simulink model "UREC_microgrid"  (R2021b)
settings: Solver=ode23tb  StartTime=0.0  StopTime=length(meters(:, 1))*SecsPerFiveMins  RelTol=1e-3
PostLoadFcn:
  | % EXCEL SCRAPING
  | 
  | [meters, timesdates] = xlsread('ExcelDataMk3.xlsx');
  | %{
  | Format:
  | No column headers
  | Times in 1st column
  | Dates in 2nd column
  | Meter data in columns 2-5
  | Times and dates will become 2 different columns of "timesdates"
  | %}
  | 
  | [pv0_power, pv0_timestamps] = xlsread('PVMk2_0axis.xlsx');
  | %{
  | Format:
  | No column headers
  | Timestamps in 1st column
  | PV output data in 2nd column
  | %}
  | 
  | [pv1_power, pv1_timestamps] = xlsread('PVMk2_1axis.xlsx');
  | %{
  | Format:
  | No column headers
  | Timestamps in 1st column
  | PV output data in 2nd column
  | %}
  | 
  | [pv2_power, pv2_timestamps] = xlsread('PVMk2_2axis.xlsx');
  | %{
  | Format:
  | No column headers
  | Timestamps in 1st column
  | PV output data in 2nd column
  | %}
  | 
  | [wind_power, wind_timestamps] = xlsread('WindMk1.xlsx');
  | %{
  | Format:
  | No column headers
  | Timestamps in 1st column
  | Wind output data in 2nd column
  | %}
  | 
  | 
  | % CONSTANTS
  | 
  | NumBatteryBanks = 1;
  | SecsPerFiveMins = 300;
  | MaxBatteryPower = 1200; %max kW for charge AND discharge of ONE Saft battery
  | TurbinekW = 1600; %The capacity of the wind turbine model, in kW
  | ThreePVs = [pv0_power, pv1_power, pv2_power]; %For easy selection with Dashboard
model workspace (MAT data in the model file):
  PVAxes = 0
  testVal = 1
  testVal1 = 1
  testVal2 = 1
undefined symbols (not defined in the file): meters, pv0_power, wind_power
libraries: simulink x6, exampleMicrogridLibrary x4, spsThreePhaseDynamicLoadLib x3, spsThreePhaseSourceLib x1, spspowerguiLib x1
settings Model: SimulationMode=accelerator  Creator=andre  LastModifiedBy=andre

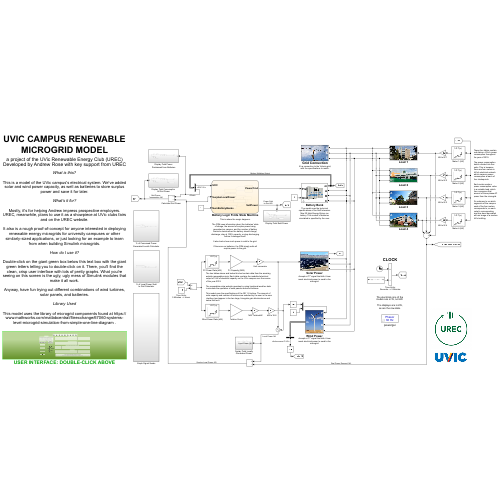
[thumbnail: Simulink's stored preview of the top-level diagram]
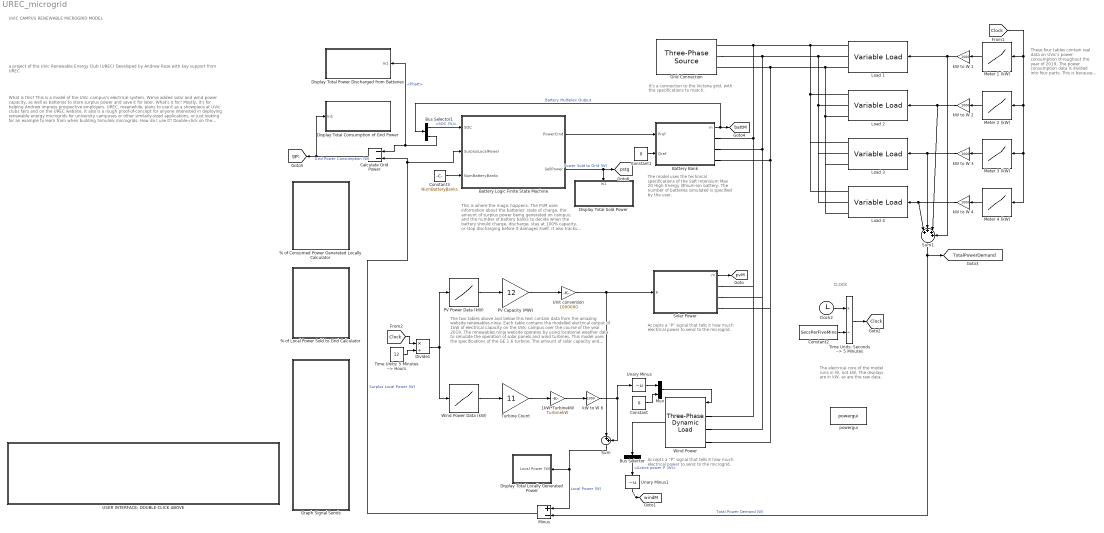
== system UREC_microgrid ==
  note: This is where the magic happens.
      |
      | The FSM uses information about the batteries' state of charge, the amount of surplus power being generated on campus, and the number of battery banks to decide when the battery should charge, discharge, stay at 100% capacity, or stop discharging before it damages itself.
      |
      | It also tracks how much power is sold to the grid.
      |
      | If there are no batteries, the FSM simply sells all surplus power to the grid.
  note: The two tables above and below this text contain data from the amazing website renewables.ninja. Each table contains the modelled electrical output of 1kW of electrical capacity on the UVic campus over the course of the year 2019.
      |
      | The renewables.ninja website operates by using locational weather data to simulate the operation of solar panels and wind turbines.
      |
      | This model uses the specifications of the GE 1.6 turbine. The amount of solar capacity and number of turbines are selected by the user in the user interface (and appear in the two large, triangular gain blocks above and below this text).
  note: Accepts a "P" signal that tells it how much electrical power to send to the microgrid.
  note: The model uses the technical specifications of the Saft Intensium Max 20 High Energy lithium-ion battery. The number of batteries simulated is specified by the user.
  note: These four tables contain real data on UVic's power consumption throughout the year of 2019.
      |
      | The power consumption data is divided into four parts. This is because there are four meters in UVic's electrical network which measure power consumption at each of four chokepoints.
      |
      | Each meter sends a power consumption value to a variable load, which then consumes that amount of three-phase AC power from the microgrid.
      |
      | It's unknown to us which segments of the campus each of the four meters corresponds to, so each meter's corresponding load has been decorated with an image of a random UVic building.
  note: UVIC CAMPUS RENEWABLE
      | MICROGRID MODEL
  note: CLOCK
  note: The electrical core of the
      | model runs in W, not kW.
      |
      | The displays are in kW,
      | as are the raw data.
  note: a project of the UVic Renewable Energy Club (UREC)
      | Developed by Andrew Rose with key support from UREC
  note: What is this?
      |
      | This is a model of the UVic campus's electrical system. We've added solar and wind power capacity, as well as batteries to store surplus power and save it for later.
      |
      | What's it for?
      |
      | Mostly, it's for helping Andrew impress prospective employers. UREC, meanwhile, plans to use it as a showpiece at UVic clubs fairs and on the UREC website.
      |
      | It also is a rough proof-of-concept for anyone interested in deploying renewable energy microgrids for university campuses or other similarly-sized applications, or just looking for an example to learn from when building Simulink microgrids.
      |
      | How do I use it?
      |
      | Double-click on the giant green box below this text box with the giant green letters telling you to double-click on it. There, you'll find the clean, crisp user interface with lots of pretty graphs. What you're seeing on this screen is the ugly, ugly mess of Simulink modules that make it all work.
      |
      | Anyway, have fun trying out different combinations of wind turbines, solar panels, and batteries.
      |
      | Library Used
      |
      | This model uses the library of microgrid components found at https://www.mathworks.com/matlabcentral/fileexchange/67060-systems-level-microgrid-simulation-from-simple-one-line-diagram .
  note: It's a connection to the Victoria grid, with the specifications to match.
  note: Accepts a "P" signal that tells it how much electrical power to send to the microgrid.
  % of Consumed Power Generated Locally Calculator : Subsystem
  % of Local Power Sold to Grid Calculator : Subsystem
  "1kW*TurbinekW " : Gain  Gain=TurbinekW
  Battery Bank : Subsystem  mask(Grid-connected Energy Storage (PQ Model)){Vn=208, Fn=60, PnomkW=MaxBatteryPower*NumBatteryBanks, kWh_Rated=2500*NumBatteryBanks, Efficiency=87.5, LimitVec=[100 10], RechargeSOC=11, Precharge=100, autoRecharge=off, Initial_kWh_pc=80, PQvec=[0 0]}
      mask prompts: Vn "Nominal L-L Voltage [Vrms]"; Fn "Nominal Frequency [Hz]"; PnomkW "Rated Power [kW]"; kWh_Rated "Rated Capacity [kWh]"; Efficiency "Overall System Efficiency [%]"; LimitVec "Upper/Lower Charge Limits [%]"; RechargeSOC "SOC to Recharge [%]"; Precharge "Recharge Rate [% of Rated Power]"; autoRecharge "Enable Auto-Recharge"; Initial_kWh_pc "Initial State-of-Charge [0-100%]"; PQvec "Initial Active/Reactive Cmds"
      mask help:
      | The energy storage block models a generic grid-connected energy storage system (ESS), most commonly a battery system. This is a system-level model that does not contain any power electronics, but is useful for load flow, phasor, and hybrid phasor-EMT simulations. The inputs to this block are the commanded active and reactive power of the ESS. The ESS is assumed to have four quadrent operation.
      |
      | For more detailed ESS models, consider the battery block in the Drives library. Consider using this PQ Model to perform load flow studies and switch to a more detailed model when full EMT studies or more advanced controls are required.
      |
      | Note: The initial active/reactive power commands must be specified for use for Load Flow analysis.
      mask init:
      | % Calculate Initial Conditions
      | Pnom = PnomkW*1e3;
      | P0 = -PQvec(1);  Q0 = -PQvec(2);
      | if abs(P0) > Pnom
      |     P0 = sign(P0)*Pnom;
      | end
      | 
      | % Calculate Q0 given Reactive Power Capability Curve
      | Qlim = sqrt(Pnom^2 - P0^2);
      | if Qlim > abs(Q0)
      |     Q0 = sign(Q0)*Qlim;
      | end
      | 
      | UpChrgLim = LimitVec(1);
      | LowChrgLim = LimitVec(2);
      | if Initial_kWh_pc > UpChrgLim && P0 < 0
      |     P0 = 0; Q0 = 0;
      | elseif Initial_kWh_pc < LowChrgLim && P0 > 0
      |     P0 = 0; Q0 = 0;
      | end
      mask DialogControl Container7 Prompt: Grid Connection Properties
      mask DialogControl Container11 Prompt: Charge/Discharge Controls
      mask DialogControl Container12 Prompt: Initial Conditions
      mask Display:
      | image('$imagefile'); % Use "Edit Image" on toolstrip to change.
      | color('black')
      | port_label('input', 1, 'Pref')
      | port_label('input', 2, 'Qref')
      | port_label('output',1,'m')
      | port_label('Rconn',1,'A')
      | port_label('Rconn',2,'B')
      | port_label('Rconn',3,'C')
  Battery Logic Finite State Machine : Stateflow chart  TreatAsAtomicUnit=on
  Bus Selector : BusSelector  OutputSignals=Active power P (W)
  Bus Selector1 : BusSelector  OutputSignals=SOC (%),Pbatt
  Calculate Grid Power : Sum  Inputs=--
  Clock2 : Clock
      settings: Decimation=1000
  Constant : Constant  Value=0
  Constant1 : Constant  Value=0
  Constant2 : Constant  Value=SecsPerFiveMins
  Constant3 : Constant  Value=NumBatteryBanks
  Display Total Consumption of Grid Power : Subsystem
  Display Total Locally Generated Power : Subsystem
  Display Total Power Discharged from Batteries : Subsystem
  Display Total Sold Power : Subsystem
      settings: PortSchema="{\"entries\":[{\"content\":{\"sides\":[{\"content\":{\"connectorIds\":[]},\"type\":\"ConnectorPlacement.EquallySpacedRectSide\",\"uuid\":\"62bf1daa-ae47-4c4c-bb60-5b8a528187ce\"},{\"content\":{\"connectorIds\":[],\"side\":\"RIGHT\"},\"type\":\"ConnectorPlacement.EquallySpacedRectSide\",\"uuid\":\"b0232ea0-dc8f-4c22-91af-b7339a0b5622\"},{\"content\":{\"connectorIds\":[\"In1\"],\"side\":\"TOP\"},\"type\":\"ConnectorPlacement.EquallySpacedRectSide\",\"uuid\":\"43a34dad-e90c-4708-b85a-e2ed5af34da1\"}]},\"type\":\"ConnectorPlacement.EquallySpacedConnector\",\"uuid\":\"1a3bae20-1562-4c93-80ee-9a5a33e73ad3\"}],\"packageUris\":[\"http://schema.mathworks.com/mf0/Connector/R2020b\"],\"version\":\"1.0\"}"
  Divide1 : Product  Inputs=*/
  Graph Signal Sends : Subsystem
  Grid Connection : spsThreePhaseSourceLib/Three-Phase Source  InternalConnection=Yg  VoltagePhases=off  Voltage=208  PhaseAngle=0  Voltage_phases=[25e3 25e3 25e3]/sqrt(3)  PhaseAngles_phases=[0 -120 +120]  Frequency=60  NonIdealSource=on  SpecifyImpedance=off  Resistance=0  Inductance=0  ShortCircuitLevel=250e6  BaseVoltage=208  XRratio=7  BusType=swing  Pref=10e3  Qref=0  Prefabc=[10e3, 10e3, 10e3]  Qrefabc=[0, 0, 0]  Qmin=-inf  Qmax=inf  mask(Three-Phase Source){}
      mask Display:
      | image('$imagefile'); % Use "Edit Image" on toolstrip to change.
      | color('white')
      | port_label('Rconn',1,'A')
      | port_label('Rconn',2,'B')
      | port_label('Rconn',3,'C')
  Load {1..4} (4 alike) : exampleMicrogridLibrary/Variable Load  Vn=208  Fn=60  PF=1  Load0=200e3  mask(Variable Load (PQ Model)){}
      settings: SourceProductName=Example Microgrid Library
      mask Display:
      | image('$imagefile'); % Use "Edit Image" on toolstrip to change.
      | color('white')
      | port_label('input',1,'Load')
      | port_label('Rconn',1,'A')
      | port_label('Rconn',2,'B')
      | port_label('Rconn',3,'C')
  Meter 1 (kW) : Lookup_n-D  NumberOfTableDimensions=1  BreakpointsForDimension1=[0:length(meters(:, 1))-1]  IndexSearchMethod=Linear search  BeginIndexSearchUsingPreviousIndexResult=on  Table=meters(:, 1)  InterpMethod=Flat  InternalRulePriority=Speed  RndMeth=Simplest  InputSameDT=on
  Meter 2 (kW) : Lookup_n-D  NumberOfTableDimensions=1  BreakpointsForDimension1=[0:length(meters(:, 1))-1]  IndexSearchMethod=Linear search  BeginIndexSearchUsingPreviousIndexResult=on  Table=meters(:, 2)  InterpMethod=Flat  InternalRulePriority=Speed  RndMeth=Simplest  InputSameDT=on
  Meter 3 (kW) : Lookup_n-D  NumberOfTableDimensions=1  BreakpointsForDimension1=[0:length(meters(:, 1))-1]  IndexSearchMethod=Linear search  BeginIndexSearchUsingPreviousIndexResult=on  Table=meters(:, 3)  InterpMethod=Flat  InternalRulePriority=Speed  RndMeth=Simplest  InputSameDT=on
  Meter 4 (kW) : Lookup_n-D  NumberOfTableDimensions=1  BreakpointsForDimension1=[0:length(meters(:, 1))-1]  IndexSearchMethod=Linear search  BeginIndexSearchUsingPreviousIndexResult=on  Table=meters(:, 4)  InterpMethod=Flat  InternalRulePriority=Speed  RndMeth=Simplest  InputSameDT=on
  Minus : Sum  Inputs=+-
  Mux : Mux  Inputs=2
  PV Capacity (MW) : Gain  Gain=12
  PV Power Data (kW) : Lookup_n-D  NumberOfTableDimensions=1  BreakpointsForDimension1=[0:length(pv0_power)-1]  IndexSearchMethod=Linear search  BeginIndexSearchUsingPreviousIndexResult=on  Table=ThreePVs(:, PVAxes+1)  InterpMethod=Flat  InternalRulePriority=Speed  RndMeth=Simplest  InputSameDT=on
  Solar Power : Subsystem  mask(Grid-Connected PV Array (PQ Model)){Vn=208, Fn=60, P0=500e3}
      mask prompts: Vn "Nominal L-L Voltage [Vrms]"; Fn "Nominal Frequency [Hz]"; P0 "Initial Power [W]"
      mask help:
      | This block models a grid-connected solar array using the Three-Phase Dynamic Load block. This is a system-level model that does not contain any power electronics, but is useful for load flow, phasor, and hybrid phasor-EMT simulations. The input to this block is the power output of the grid connected PV array, not irradiance.
      |
      | For more detailed PV models, consider the PV Array block in the Renewables library. Consider using this PQ Model to perform load flow studies and switch to a more detailed model when full EMT studies are required.
      |
      | Note: The array power must be specified for use for Load Flow analysis.
      mask init:
      | % P0 = Irr0*TotalArea*Efficiency/100;
      | P0 = -P0;
      mask Display:
      | image(imread('PV_Farm.jpg'))
      | color('white')
      | port_label('input',1,'P')
      | port_label('output',1,'m')
      | port_label('Rconn',1,'A')
      | port_label('Rconn',2,'B')
      | port_label('Rconn',3,'C')
  Sum : Sum  Inputs=|++
  Sum1 : Sum  Inputs=|++++
  Time Units: 5 Minutes --> Hours : Constant  Value=12
  Time Units: Seconds --> 5 Minutes : Product  Inputs=*/
  Turbine Count : Gain  Gain=11
  USER INTERFACE: DOUBLE-CLICK ABOVE : Subsystem
  Unary Minus : UnaryMinus
  Unary Minus1 : UnaryMinus
  Unit conversion : Gain  Gain=1000000
  Wind Power : spsThreePhaseDynamicLoadLib/Three-Phase Dynamic Load  NominalVoltage=[208 60 ]  ActiveReactivePowers=[50e6 25e6]  PositiveSequence=[0.994 -11.8]  ExternalControl=on  NpNq=[1.3 2]  TimeConstants="[0  0  0  0]"  MinimumVoltage=0.7  Tfilter=1e-2  LoadFlowParameters=[4,0,0,0,0]  mask(Three-Phase Dynamic Load){}
      settings: SourceProductBaseCode=PS
      mask Display:
      | image('$imagefile'); % Use "Edit Image" on toolstrip to change.
      | color('white')
      | port_label('input',1,'P')
      | port_label('output',1,'m')
      | port_label('Lconn',1,'A')
      | port_label('Lconn',2,'B')
      | port_label('Lconn',3,'C')
  Wind Power Data (kW) : Lookup_n-D  NumberOfTableDimensions=1  BreakpointsForDimension1=[0:length(wind_power)-1]  IndexSearchMethod=Linear search  BeginIndexSearchUsingPreviousIndexResult=on  Table=wind_power(:)  InterpMethod=Flat  InternalRulePriority=Speed  RndMeth=Simplest  InputSameDT=on
  kW to W {1..4,6} (5 alike) : Gain  Gain=1000
  powergui : spspowerguiLib/powergui  Priority=1  SimulationMode=Phasor  SampleTime=1e-4  frequency=60  Iterations=50  frequencyindice=60  Pbase=100e6  ErrMax=0.0001  UnitsV=kV  UnitsW=MW  buscounter=3  FunctionMessages=off  echomessages=off  EnableUseOfTLC=off  CurrentSourceSwitches=off  DisableSnubberDevices=off  DisableRonSwitches=off  DisableVfSwitches=off  DisplayEquations=off  AutomaticDiscreteSolvers=off  SolverType=Tustin/Backward Euler (TBE)  Interpol=off  ExternalGateDelay=off  methode=off  Ts=100  x0status=blocks  SPID=on  SwTol=0  HookPort=off  NonlinearTolerance=1e-4  nMaxIteration=100  ContinueOnMaxIteration=off  RestoreLinks=warning  ResistiveCurrentMeasurement=off  Frange=[0:2:500]  Ylog=off  Xlog=on  ShowGrid=off  save=off  variable=ZData  structure=0  ZoomFFT=off  StartTime=0.0  cycles=1  DisplayStyle=1  fundamental=60  FreqAxis=off  MaxFrequency=1000  frequencyindicesteady=1  RmsSteady=1  display=off
  tag scope: Clock=global, TotalPowerDemand=global, battM=global, gpc=global, pstg=global, pvM=global, windM=global
  wires:
  [Clock] -> Meter 4 (kW)/1, Meter 3 (kW)/1, Meter 2 (kW)/1, Meter 1 (kW)/1
  Meter 2 (kW)/1 -> kW to W 2/1
  Meter 3 (kW)/1 -> kW to W 3/1
  Meter 4 (kW)/1 -> kW to W 4/1
  Time Units: 5 Minutes --> Hours/1 -> Divide1/2
  [Clock] -> Divide1/1
  Divide1/1 -> Wind Power Data (kW)/1, PV Power Data (kW)/1
  PV Power Data (kW)/1 -> PV Capacity (MW)/1
  Solar Power/1(m) -> [pvM]
  Wind Power Data (kW)/1 -> Turbine Count/1
  Constant/1 -> Mux/2
  Mux/1 -> Wind Power/1
  Unary Minus/1 -> Mux/1
  Wind Power/1 -> Bus Selector/1
  Bus Selector/1 -> Unary Minus1/1  "<Active power P (W)>"
  Unary Minus1/1 -> [windM]
  Sum1/1 -> Minus/2, [TotalPowerDemand]  "Total Power Demand (W)"
  Sum/1 -> Minus/1, Display Total Locally Generated Power/1(Local Power (W))  "Local Power (W)"
  Minus/1 -> Calculate Grid Power/2, Battery Logic Finite State Machine/2(SurplusLocalPower)  "Surplus Local Power (W)"
  Clock2/1 -> Time Units: Seconds --> 5 Minutes/1
  Constant2/1 -> Time Units: Seconds --> 5 Minutes/2
  Time Units: Seconds --> 5 Minutes/1 -> [Clock]
  Constant1/1 -> Battery Bank/2(Qref)
  Battery Logic Finite State Machine/1(PowerCmd) -> Battery Bank/1(Pref)
  Battery Bank/1(m) -> [battM], Bus Selector1/1  "Battery Multiplex Output"
  Bus Selector1/1 -> Battery Logic Finite State Machine/1(SOC)  "<SOC (%)>"
  Meter 1 (kW)/1 -> kW to W 1/1
  kW to W 3/1 -> Load 3/1, Sum1/2
  Unit conversion/1 -> Solar Power/1(P), Sum/1
  kW to W 6/1 -> Unary Minus/1, Sum/2
  kW to W 1/1 -> Sum1/4, Load 1/1
  kW to W 2/1 -> Load 2/1, Sum1/3
  kW to W 4/1 -> Load 4/1, Sum1/1
  "1kW*TurbinekW "/1 -> kW to W 6/1
  PV Capacity (MW)/1 -> Unit conversion/1
  Turbine Count/1 -> "1kW*TurbinekW "/1
  Bus Selector1/2 -> Calculate Grid Power/1, Display Total Power Discharged from Batteries/1(In1)  "<Pbatt>"
  Battery Logic Finite State Machine/2(SellPower) -> Display Total Sold Power/1(In1), [pstg]  "Power Sold to Grid (W)"
  Calculate Grid Power/1 -> [gpc], Display Total Consumption of Grid Power/1(In1)  "Grid Power Consumption (W)"
  Constant3/1 -> Battery Logic Finite State Machine/3(NumBatteryBanks)
  connections:
  Load 1/RConn1 -- Load 4/RConn1 -- Load 3/RConn1 -- Load 2/RConn1 -- Solar Power/RConn1 -- Wind Power/LConn1 -- Battery Bank/RConn1 -- Grid Connection/RConn1
  Load 1/RConn2 -- Load 4/RConn2 -- Load 3/RConn2 -- Load 2/RConn2 -- Solar Power/RConn2 -- Wind Power/LConn2 -- Battery Bank/RConn2 -- Grid Connection/RConn2
  Load 1/RConn3 -- Load 4/RConn3 -- Load 3/RConn3 -- Load 2/RConn3 -- Solar Power/RConn3 -- Wind Power/LConn3 -- Battery Bank/RConn3 -- Grid Connection/RConn3

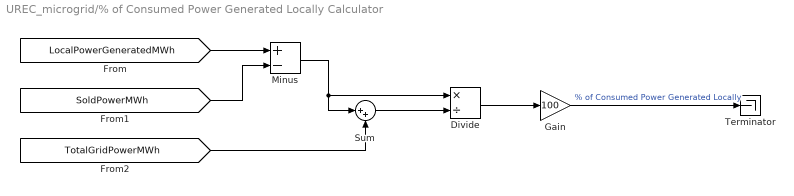
== system UREC_microgrid/% of Consumed Power Generated Locally Calculator ==
  Divide : Product  Inputs=*/
  Gain : Gain  Gain=100
  Minus : Sum  Inputs=+-
  Sum : Sum  Inputs=|++
  Terminator : Terminator
  wires:
  [LocalPowerGeneratedMWh] -> Minus/1
  [SoldPowerMWh] -> Minus/2
  Minus/1 -> Divide/1, Sum/1
  [TotalGridPowerMWh] -> Sum/2
  Sum/1 -> Divide/2
  Gain/1 -> Terminator/1  "% of Consumed Power Generated Locally"
  Divide/1 -> Gain/1

== system UREC_microgrid/% of Local Power Sold to Grid Calculator ==
  Divide : Product  Inputs=*/
  Gain : Gain  Gain=100
  Terminator : Terminator
  wires:
  [LocalPowerGeneratedMWh] -> Divide/2
  [SoldPowerMWh] -> Divide/1
  Divide/1 -> Gain/1
  Gain/1 -> Terminator/1  "% of Local Power Sold to Grid"

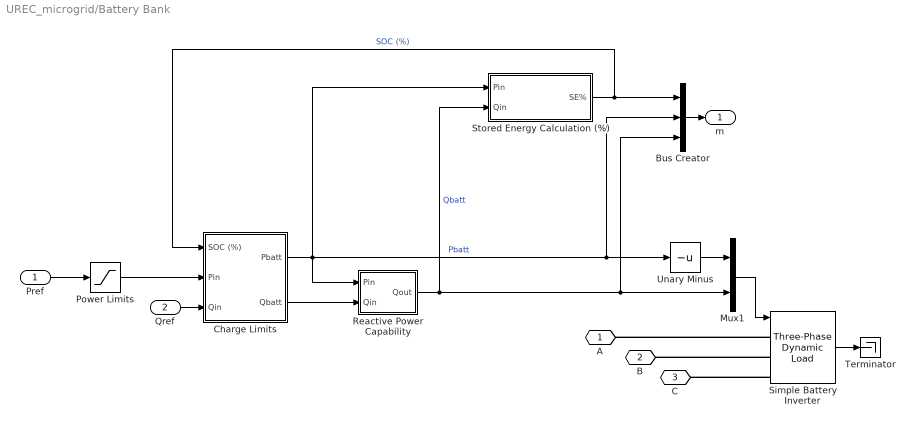
== system UREC_microgrid/Battery Bank ==
  Pref : Inport
  Qref : Inport  Port=2
  Bus Creator : BusCreator  Inputs=3
  Charge Limits : Subsystem
  Mux1 : Mux  Inputs=2
  Power Limits : Saturate  UpperLimit=Pnom  LowerLimit=-Pnom
  Reactive Power Capability : Subsystem
  Simple Battery Inverter : spsThreePhaseDynamicLoadLib/Three-Phase Dynamic Load  NominalVoltage=[Vn Fn]  ActiveReactivePowers=[-500000 -3.38813e-13]  PositiveSequence=[0.999844 -0.0038635]  ExternalControl=on  NpNq=[1.3 2]  TimeConstants="[0  0  0  0]"  MinimumVoltage=0.7  Tfilter=1e-2  LoadFlowParameters=[4,0,0,0,0]
      settings: SourceProductBaseCode=PS
  Stored Energy Calculation (%) : Subsystem
  Terminator : Terminator
  Unary Minus : UnaryMinus
  A : PMIOPort  Side=Right
  B : PMIOPort  Port=2  Side=Right
  C : PMIOPort  Port=3  Side=Right
  m : Outport  VectorParamsAs1DForOutWhenUnconnected=off
  wires:
  Charge Limits/2(Qbatt) -> Reactive Power Capability/2(Qin)
  Qref/1 -> Charge Limits/3(Qin)
  Power Limits/1 -> Charge Limits/2(Pin)
  Charge Limits/1(Pbatt) -> Reactive Power Capability/1(Pin), Unary Minus/1, Bus Creator/2, Stored Energy Calculation (%)/1(Pin)  "Pbatt"
  Stored Energy Calculation (%)/1(SE%) -> Bus Creator/1, Charge Limits/1(SOC (%))  "SOC (%)"
  Bus Creator/1 -> m/1
  Pref/1 -> Power Limits/1
  Reactive Power Capability/1(Qout) -> Mux1/2, Bus Creator/3, Stored Energy Calculation (%)/2(Qin)  "Qbatt"
  Simple Battery Inverter/1 -> Terminator/1
  Mux1/1 -> Simple Battery Inverter/1
  Unary Minus/1 -> Mux1/1
  connections:
  Simple Battery Inverter/LConn1 -- A/RConn1
  Simple Battery Inverter/LConn3 -- C/RConn1
  Simple Battery Inverter/LConn2 -- B/RConn1

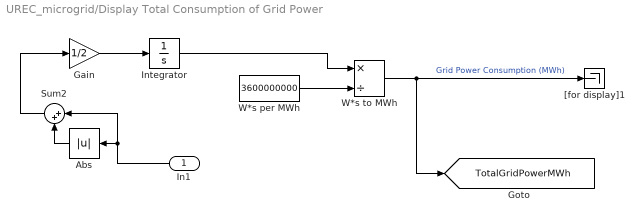
== system UREC_microgrid/Display Total Consumption of Grid Power ==
  In1 : Inport
  Abs : Abs
  Gain : Gain  Gain=1/2
  Integrator : Integrator
  Sum2 : Sum  Inputs=|++
  W*s per MWh : Constant  Value=3600000000
  W*s to MWh : Product  Inputs=*/
  "[for display]1" : Terminator
  tag scope: TotalGridPowerMWh=global
  wires:
  Abs/1 -> Sum2/2
  W*s per MWh/1 -> W*s to MWh/2
  W*s to MWh/1 -> [TotalGridPowerMWh], "[for display]1"/1  "Grid Power Consumption (MWh)"
  In1/1 -> Sum2/1, Abs/1
  Integrator/1 -> W*s to MWh/1
  Sum2/1 -> Gain/1
  Gain/1 -> Integrator/1

== system UREC_microgrid/Display Total Locally Generated Power ==
  Local Power (W) : Inport
  Integrate1 : Integrator
  W*s per MWh1 : Constant  Value=3600000000
  W*s to MWh1 : Product  Inputs=*/
  "[for display]2" : Terminator
  tag scope: LocalPowerGeneratedMWh=global
  wires:
  W*s to MWh1/1 -> [LocalPowerGeneratedMWh], "[for display]2"/1  "Local Power Generated (MWh)"
  W*s per MWh1/1 -> W*s to MWh1/2
  Integrate1/1 -> W*s to MWh1/1
  Local Power (W)/1 -> Integrate1/1

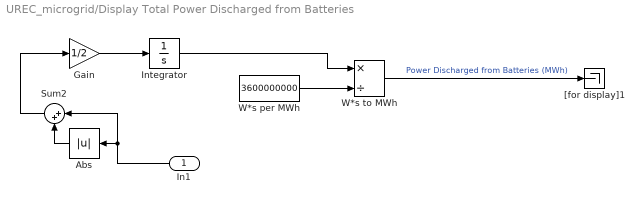
== system UREC_microgrid/Display Total Power Discharged from Batteries ==
  In1 : Inport
  Abs : Abs
  Gain : Gain  Gain=1/2
  Integrator : Integrator
  Sum2 : Sum  Inputs=|++
  W*s per MWh : Constant  Value=3600000000
  W*s to MWh : Product  Inputs=*/
  "[for display]1" : Terminator
  wires:
  Abs/1 -> Sum2/2
  W*s per MWh/1 -> W*s to MWh/2
  W*s to MWh/1 -> "[for display]1"/1  "Power Discharged from Batteries (MWh)"
  In1/1 -> Sum2/1, Abs/1
  Integrator/1 -> W*s to MWh/1
  Sum2/1 -> Gain/1
  Gain/1 -> Integrator/1

== system UREC_microgrid/Display Total Sold Power ==
  In1 : Inport
  Integrate : Integrator
  W*s per MWh : Constant  Value=3600000000
  W*s to MWh : Product  Inputs=*/
  "[for display]" : Terminator
  tag scope: SoldPowerMWh=global
  wires:
  Integrate/1 -> W*s to MWh/1
  W*s per MWh/1 -> W*s to MWh/2
  W*s to MWh/1 -> [SoldPowerMWh], "[for display]"/1  "Local Power Sold to Grid (MWh)"
  In1/1 -> Integrate/1

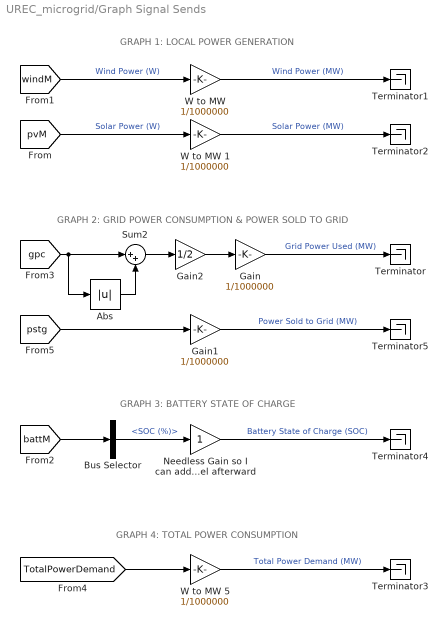
== system UREC_microgrid/Graph Signal Sends ==
  note: GRAPH 1: LOCAL POWER GENERATION
  note: GRAPH 4: TOTAL POWER CONSUMPTION
  note: GRAPH 3: BATTERY STATE OF CHARGE
  note: GRAPH 2: GRID POWER CONSUMPTION & POWER SOLD TO GRID
  Abs : Abs
  Bus Selector : BusSelector  OutputSignals=SOC (%)
  Gain : Gain  Gain=1/1000000
  Gain1 : Gain  Gain=1/1000000
  Gain2 : Gain  Gain=1/2
  Needless Gain so I can add a new label afterward : Gain
  Sum2 : Sum  Inputs=|++
  Terminator{,1..5} (6 alike) : Terminator
  W to MW : Gain  Gain=1/1000000
  W to MW 1 : Gain  Gain=1/1000000
  W to MW 5 : Gain  Gain=1/1000000
  wires:
  [TotalPowerDemand] -> W to MW 5/1
  [pvM] -> W to MW 1/1  "Solar Power (W)"
  [windM] -> W to MW/1  "Wind Power (W)"
  [battM] -> Bus Selector/1
  Bus Selector/1 -> Needless Gain so I can add a new label afterward/1  "<SOC (%)>"
  Needless Gain so I can add a new label afterward/1 -> Terminator4/1  "Battery State of Charge (SOC)"
  W to MW 5/1 -> Terminator3/1  "Total Power Demand (MW)"
  W to MW/1 -> Terminator1/1  "Wind Power (MW)"
  W to MW 1/1 -> Terminator2/1  "Solar Power (MW)"
  Gain/1 -> Terminator/1  "Grid Power Used (MW)"
  Gain1/1 -> Terminator5/1  "Power Sold to Grid (MW)"
  [pstg] -> Gain1/1
  Sum2/1 -> Gain2/1
  Abs/1 -> Sum2/2
  Gain2/1 -> Gain/1
  [gpc] -> Sum2/1, Abs/1

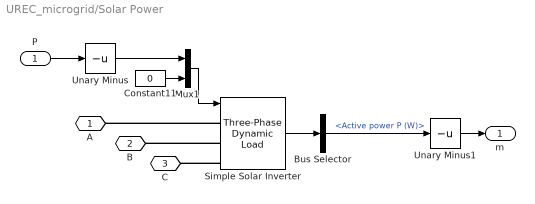
== system UREC_microgrid/Solar Power ==
  P : Inport
  Bus Selector : BusSelector  OutputSignals=Active power P (W)
  Constant11 : Constant  Value=0
  Mux1 : Mux  Inputs=2
  Simple Solar Inverter : spsThreePhaseDynamicLoadLib/Three-Phase Dynamic Load  NominalVoltage=[Vn Fn]  ActiveReactivePowers=[-250000 -3.38813e-13]  PositiveSequence=[0.999844 -0.0038635]  ExternalControl=on  NpNq=[1.3 2]  TimeConstants="[0  0  0  0]"  MinimumVoltage=0.7  Tfilter=1e-2  LoadFlowParameters=[4,0,0,0,0]
      settings: SourceProductBaseCode=PS
  Unary Minus : UnaryMinus
  Unary Minus1 : UnaryMinus
  A : PMIOPort  Side=Right
  B : PMIOPort  Port=2  Side=Right
  C : PMIOPort  Port=3  Side=Right
  m : Outport  VectorParamsAs1DForOutWhenUnconnected=off
  wires:
  P/1 -> Unary Minus/1
  Unary Minus/1 -> Mux1/1
  Mux1/1 -> Simple Solar Inverter/1
  Constant11/1 -> Mux1/2
  Simple Solar Inverter/1 -> Bus Selector/1
  Bus Selector/1 -> Unary Minus1/1  "<Active power P (W)>"
  Unary Minus1/1 -> m/1
  connections:
  Simple Solar Inverter/LConn2 -- B/RConn1
  Simple Solar Inverter/LConn3 -- C/RConn1
  Simple Solar Inverter/LConn1 -- A/RConn1

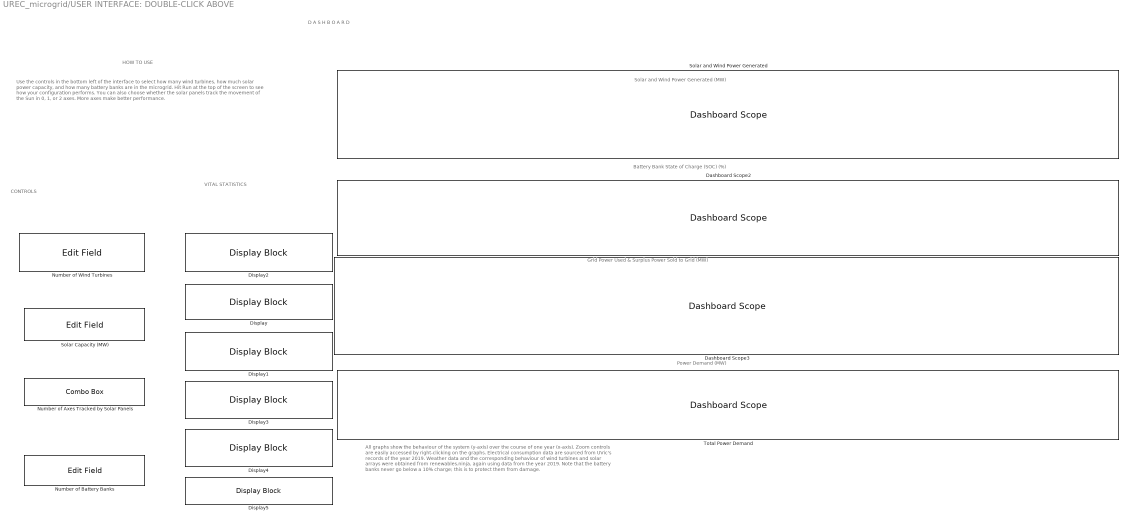
== system UREC_microgrid/USER INTERFACE: DOUBLE-CLICK ABOVE ==
  note: Use the controls in the bottom left of the interface to select how many wind turbines, how much solar power capacity, and how many battery banks are in the microgrid. Hit Run at the top of the screen to see how your configuration performs.
      |
      | You can also choose whether the solar panels track the movement of the Sun in 0, 1, or 2 axes. More axes make better performance.
  note: HOW TO USE
  note: VITAL
      | STATISTICS
  note: D A S H B O A R D
  note: All graphs show the behaviour of the system (y-axis) over the course of one year (x-axis).
      | Zoom controls are easily accessed by right-clicking on the graphs.
      | Electrical consumption data are sourced from UVic's records of the year 2019.
      | Weather data and the corresponding behaviour of wind turbines and solar arrays were obtained from renewables.ninja, again using data from the year 2019.
      | Note that the battery banks never go below a 10% charge; this is to protect them from damage.
  note: Solar and Wind Power Generated (MW)
  note: Power Demand (MW)
  note: Battery Bank State of Charge (SOC) (%)
  note: Grid Power Used & Surplus Power Sold to Grid (MW)
  note: CONTROLS
  Dashboard Scope2 : DashboardScope  ShowInitialText=off  TimeSpan=31622400  LegendPosition=Hide  UpdateMode=Scroll
      settings: TickLabels=Y-Axis
  Dashboard Scope3 : DashboardScope  ShowInitialText=off  TimeSpan=31622400  UpdateMode=Scroll
      settings: TickLabels=Y-Axis
  Display{,1..3} (4 alike) : DisplayBlock  LabelPosition=Bottom  Format=Custom  Transparency=1  FormatString=%.2f
  Display4 : DisplayBlock  LabelPosition=Bottom  Format=Custom  Transparency=1  FormatString=%.2f%%
  Display5 : DisplayBlock  LabelPosition=Bottom  Format=Custom  Transparency=1  FormatString=%.2f%%
  Number of Axes Tracked by Solar Panels : ComboBox  LabelPosition=Hide  SelectedLabel=0
      settings: Values={{'0', '1', '2'}, [0 1 2]}
  Number of Battery Banks : EditField  Tag=Number of Battery Banks  LabelPosition=Hide  ShowInitialText=on  Alignment=Center
  Number of Wind Turbines : EditField  LabelPosition=Hide  ShowInitialText=on  Alignment=Center
  Solar Capacity (MW) : EditField  Tag=Solar Capacity (MW)  LabelPosition=Hide  ShowInitialText=on  Alignment=Center
  Solar and Wind Power Generated : DashboardScope  ShowInitialText=off  TimeSpan=31622400  UpdateMode=Scroll
      settings: TickLabels=Y-Axis
  Total Power Demand : DashboardScope  ShowInitialText=off  TimeSpan=31622400  LegendPosition=Hide  UpdateMode=Scroll
      settings: TickLabels=Y-Axis

== system UREC_microgrid/Battery Bank/Charge Limits ==
  SOC (%) : Inport
  Pin : Inport  Port=2
  Qin : Inport  Port=3
  Overcharge Check : Subsystem
  Undercharge Check : Subsystem
  Pbatt : Outport  VectorParamsAs1DForOutWhenUnconnected=off
  Qbatt : Outport  Port=2  VectorParamsAs1DForOutWhenUnconnected=off
  wires:
  SOC (%)/1 -> Overcharge Check/1(SOC (%)), Undercharge Check/1(SOC (%))
  Undercharge Check/2(Qout) -> Qbatt/1
  Pin/1 -> Overcharge Check/2(Pin)
  Overcharge Check/1(Pout) -> Undercharge Check/2(Pin)
  Qin/1 -> Overcharge Check/3(Qin)
  Undercharge Check/1(Pout) -> Pbatt/1  "Pbatt"
  Overcharge Check/2(Qout) -> Undercharge Check/3(Qin)

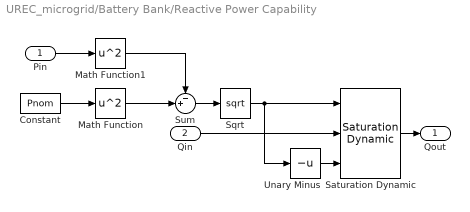
== system UREC_microgrid/Battery Bank/Reactive Power Capability ==
  Pin : Inport
  Qin : Inport  Port=2
  Constant : Constant  Value=Pnom
  Math Function : Math  Operator=square  SignedPower=on  SaturateOnIntegerOverflow=on
  Math Function1 : Math  Operator=square  SignedPower=on  SaturateOnIntegerOverflow=on
  Saturation Dynamic : simulink/Discontinuities/Saturation Dynamic  OutMin=[]  OutMax=[]  OutDataTypeStr=Inherit: Same as second input  OutDataType=fixdt(1, 16)  OutScaling=2^-10  DoSatur=off
  Sqrt : Sqrt  SaturateOnIntegerOverflow=on
  Sum : Sum  Inputs=-+|
  Unary Minus : UnaryMinus
  Qout : Outport  VectorParamsAs1DForOutWhenUnconnected=off
  wires:
  Sqrt/1 -> Saturation Dynamic/1, Unary Minus/1
  Math Function1/1 -> Sum/1
  Math Function/1 -> Sum/2
  Constant/1 -> Math Function/1
  Sum/1 -> Sqrt/1
  Unary Minus/1 -> Saturation Dynamic/3
  Saturation Dynamic/1 -> Qout/1
  Pin/1 -> Math Function1/1
  Qin/1 -> Saturation Dynamic/2

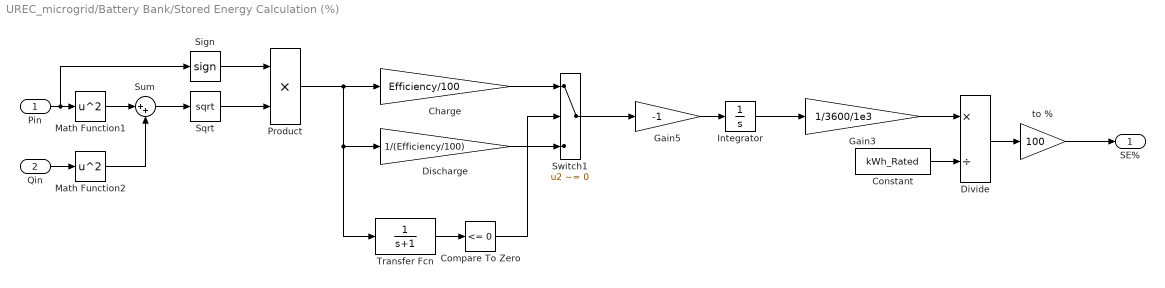
== system UREC_microgrid/Battery Bank/Stored Energy Calculation (%) ==
  Pin : Inport
  Qin : Inport  Port=2
  Charge : Gain  Gain=Efficiency/100
  Compare To Zero : simulink/Logic and Bit Operations/Compare To Zero  relop=<=  OutDataTypeStr=boolean
  Constant : Constant  Value=kWh_Rated
  Discharge : Gain  Gain=1/(Efficiency/100)
  Divide : Product  Inputs=*/
  Gain3 : Gain  Gain=1/3600/1e3
  Gain5 : Gain  Gain=-1
  Integrator : Integrator  InitialCondition=(Initial_kWh_pc/100)*kWh_Rated*3600*1e3
  Math Function1 : Math  Operator=square  SignedPower=on  SaturateOnIntegerOverflow=on
  Math Function2 : Math  Operator=square  SignedPower=on  SaturateOnIntegerOverflow=on
  Product : Product
  Sign : Signum
  Sqrt : Sqrt  SaturateOnIntegerOverflow=on
  Sum : Sum  Inputs=|++
  Switch1 : Switch  Criteria=u2 ~= 0
  Transfer Fcn : TransferFcn  Denominator=[1 1]
  to % : Gain  Gain=100
  SE% : Outport  VectorParamsAs1DForOutWhenUnconnected=off
  wires:
  Sign/1 -> Product/1
  Sqrt/1 -> Product/2
  Sum/1 -> Sqrt/1
  Math Function2/1 -> Sum/2
  Math Function1/1 -> Sum/1
  Qin/1 -> Math Function2/1
  Pin/1 -> Math Function1/1, Sign/1
  Product/1 -> Transfer Fcn/1, Discharge/1, Charge/1
  Discharge/1 -> Switch1/3
  Gain5/1 -> Integrator/1
  to %/1 -> SE%/1
  Transfer Fcn/1 -> Compare To Zero/1
  Switch1/1 -> Gain5/1
  Gain3/1 -> Divide/1
  Constant/1 -> Divide/2
  Charge/1 -> Switch1/1
  Divide/1 -> to %/1
  Compare To Zero/1 -> Switch1/2
  Integrator/1 -> Gain3/1

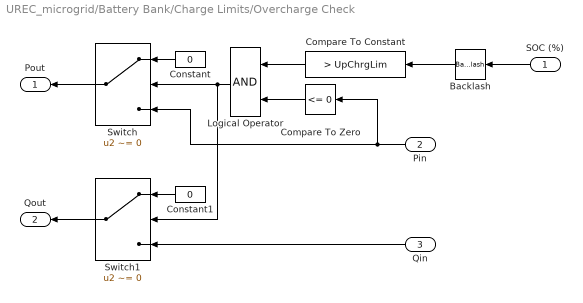
== system UREC_microgrid/Battery Bank/Charge Limits/Overcharge Check ==
  SOC (%) : Inport
  Pin : Inport  Port=2
  Qin : Inport  Port=3
  Backlash : Backlash  BacklashWidth=1e-3  InitialOutput=Initial_kWh_pc  ZeroCross=off
  Compare To Constant : simulink/Logic and Bit Operations/Compare To Constant  relop=>  const=UpChrgLim  OutDataTypeStr=boolean
  Compare To Zero : simulink/Logic and Bit Operations/Compare To Zero  relop=<=  OutDataTypeStr=boolean
  Constant : Constant  Value=0
  Constant1 : Constant  Value=0
  Logical Operator : Logic  AllPortsSameDT=off  OutDataTypeStr=boolean
  Switch : Switch  Criteria=u2 ~= 0
  Switch1 : Switch  Criteria=u2 ~= 0
  Pout : Outport  VectorParamsAs1DForOutWhenUnconnected=off
  Qout : Outport  Port=2  VectorParamsAs1DForOutWhenUnconnected=off
  wires:
  Backlash/1 -> Compare To Constant/1
  Switch1/1 -> Qout/1
  Constant1/1 -> Switch1/1
  Qin/1 -> Switch1/3
  Compare To Zero/1 -> Logical Operator/2
  Switch/1 -> Pout/1
  Pin/1 -> Switch/3, Compare To Zero/1
  SOC (%)/1 -> Backlash/1
  Constant/1 -> Switch/1
  Logical Operator/1 -> Switch/2, Switch1/2
  Compare To Constant/1 -> Logical Operator/1

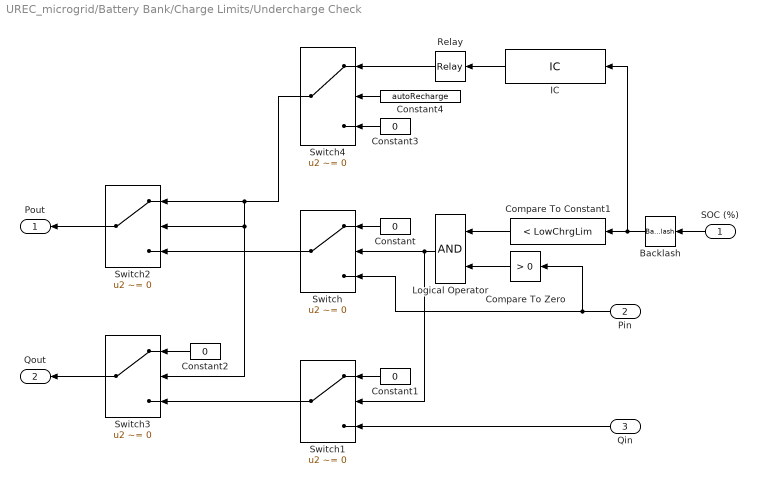
== system UREC_microgrid/Battery Bank/Charge Limits/Undercharge Check ==
  SOC (%) : Inport
  Pin : Inport  Port=2
  Qin : Inport  Port=3
  Backlash : Backlash  BacklashWidth=1e-3  InitialOutput=Initial_kWh_pc  ZeroCross=off
  Compare To Constant1 : simulink/Logic and Bit Operations/Compare To Constant  relop=<  const=LowChrgLim  OutDataTypeStr=boolean
  Compare To Zero : simulink/Logic and Bit Operations/Compare To Zero  relop=>  OutDataTypeStr=boolean
  Constant{,1..3} (4 alike) : Constant  Value=0
  Constant4 : Constant  Value=autoRecharge
  IC : InitialCondition  Value=RechargeSOC
  Logical Operator : Logic  AllPortsSameDT=off  OutDataTypeStr=boolean
  Relay : Relay  OnSwitchValue=RechargeSOC  OffSwitchValue=LowChrgLim  OnOutputValue=0  OffOutputValue=-Precharge/100*Pnom
  Switch{,1..4} (5 alike) : Switch  Criteria=u2 ~= 0
  Pout : Outport  VectorParamsAs1DForOutWhenUnconnected=off
  Qout : Outport  Port=2  VectorParamsAs1DForOutWhenUnconnected=off
  wires:
  Constant4/1 -> Switch4/2
  Constant3/1 -> Switch4/3
  Relay/1 -> Switch4/1
  Constant2/1 -> Switch3/1
  Switch1/1 -> Switch3/3
  Switch3/1 -> Qout/1
  Switch2/1 -> Pout/1
  Switch/1 -> Switch2/3
  IC/1 -> Relay/1
  Switch4/1 -> Switch3/2, Switch2/2, Switch2/1
  Backlash/1 -> Compare To Constant1/1, IC/1
  Qin/1 -> Switch1/3
  Constant1/1 -> Switch1/1
  Compare To Constant1/1 -> Logical Operator/1
  Logical Operator/1 -> Switch1/2, Switch/2
  Constant/1 -> Switch/1
  SOC (%)/1 -> Backlash/1
  Pin/1 -> Compare To Zero/1, Switch/3
  Compare To Zero/1 -> Logical Operator/2

== stateflow chart UREC_microgrid/Battery Logic Finite State Machine ==
  state NoBatteriesSellPower
    % If there are no batteries, sell all surplus power to the grid.
    entry:
    PowerCmd=0;
    during:
    SellPower=SurplusLocalPower;
  state NoBatteriesFork
    % A safety state that processes whether the user has specified zero or nonzero battery
    % banks.
    entry:
    PowerCmd=0;
    SellPower=0;
  state NoBatteriesSellNothing
    % If there are no batteries and no surplus,
    % there's nothing to sell.
    entry:
    PowerCmd=0;
    during:
    SellPower=0;
  state Charging
    % Do this whenever more power is being generated than demanded.
    % (Unless the battery is full or the surplus is more than the battery can accept.)
    entry:
    SellPower = 0;
    during:
    PowerCmd = -1*min(MaxBatteryPower*1000*NumBatteryBanks, SurplusLocalPower);
    % *1000 because units (W, kW)
  state SellSurplus
    % If the battery is full and there's a surplus of local power,
    % sell the surplus back to the grid.
    entry:
    PowerCmd = 0;
    during:
    SellPower = SurplusLocalPower;
  state Overload
    % Do this when the batteries are not full and there's such a huge surplus of power that the
    % batteries can't charge fast enough to accept it.
    % Charge the batteries as fast as possible; sell the remaining surplus to the grid.
    entry:
    PowerCmd = -1000*MaxBatteryPower*NumBatteryBanks;
    during:
    SellPower = SurplusLocalPower - 1000*MaxBatteryPower*NumBatteryBanks;
    % *1000 because units (W, kW)
  state KeepTenPercent
    % Don't discharge beyond 10%.
    % This state prevents damage to the battery.
    entry:
    PowerCmd = 0;
    SellPower=0;
  state Discharging
    % Do this whenever more power is being demanded than generated.
    % (Unless the battery is about to dip below 10% charge.)
    entry:
    SellPower = 0;
    during:
    PowerCmd = min(MaxBatteryPower*1000*NumBatteryBanks, -1*SurplusLocalPower);
    % *1000 because units (W, kW)
  NoBatteriesFork -> NoBatteriesSellPower [order 2] : [NumBatteryBanks<=0 && SurplusLocalPower>0]
  NoBatteriesSellPower -> NoBatteriesSellNothing : [SurplusLocalPower<=0]
  NoBatteriesSellNothing -> NoBatteriesSellPower : [SurplusLocalPower>0]
  (default) -> NoBatteriesFork
  NoBatteriesFork -> NoBatteriesSellNothing [order 3] : [NumBatteryBanks<=0 && SurplusLocalPower<=0]
  NoBatteriesFork -> Charging [order 1] : [NumBatteryBanks>0]
  Discharging -> Charging [order 2] : [SurplusLocalPower>0]
  Charging -> Discharging [order 3] : [SurplusLocalPower<0]
  Charging -> SellSurplus [order 1] : [(SurplusLocalPower>0) && (SOC>=100)]
  KeepTenPercent -> Charging [order 2] : [SurplusLocalPower>0]
  Charging -> Overload [order 2] : [SurplusLocalPower>1000*MaxBatteryPower*NumBatteryBanks]
  Overload -> Charging [order 3] : [(SurplusLocalPower>0) && (SurplusLocalPower<1000*MaxBatteryPower*NumBatteryBanks) && (SOC<100)]
  Overload -> SellSurplus [order 1] : [(SurplusLocalPower>0) && (SOC>=100)]
  SellSurplus -> Discharging : [SurplusLocalPower<0]
  KeepTenPercent -> Overload [order 1] : [SurplusLocalPower>1000*MaxBatteryPower*NumBatteryBanks]
  Discharging -> Overload [order 1] : [SurplusLocalPower>1000*MaxBatteryPower*NumBatteryBanks]
  Discharging -> KeepTenPercent [order 3] : [SOC<=10]
  Overload -> Discharging [order 2] : [SurplusLocalPower<=0]
  data: MaxBatteryPower parameter; PowerCmd output; SellPower output; SOC input; SurplusLocalPower input; NumBatteryBanks input
